simulink model "DiscreteStateSpace"  (R2017a)
settings: Solver=FixedStepAuto  StartTime=0.0  StopTime=10.0  FixedStep=sys.Ts  RelTol=1e-3
undefined symbols (not defined in the file): sys
settings Model: Creator=bhannigan  LastModifiedBy=bhannigan

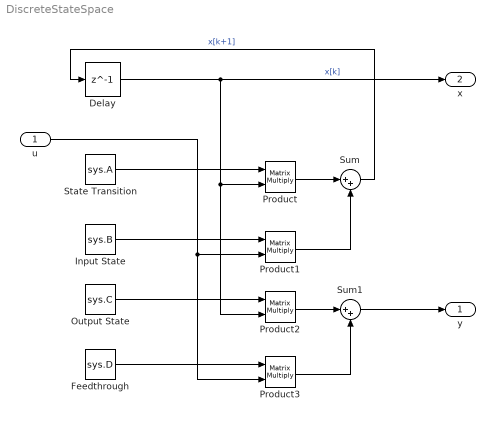
== system DiscreteStateSpace ==
  u : Inport
  Delay : Delay  DelayLength=1  InitialCondition=0
  Feedthrough : Constant  Value=sys.D  VectorParams1D=off
  Input State : Constant  Value=sys.B  VectorParams1D=off
  Output State : Constant  Value=sys.C  VectorParams1D=off
  Product{,1..3} (4 alike) : Product  Multiplication=Matrix(*)
  State Transition : Constant  Value=sys.A  VectorParams1D=off
  Sum : Sum  Inputs=|++
  Sum1 : Sum  Inputs=|++
  y : Outport
  x : Outport  Port=2
  wires:
  Delay/1 -> Product/2, Product2/2, x/1  "x[k]"
  Product/1 -> Sum/1
  Product1/1 -> Sum/2
  Sum/1 -> Delay/1  "x[k+1]"
  Product2/1 -> Sum1/1
  Product3/1 -> Sum1/2
  Sum1/1 -> y/1
  u/1 -> Product1/2, Product3/2
  Feedthrough/1 -> Product3/1
  Output State/1 -> Product2/1
  Input State/1 -> Product1/1
  State Transition/1 -> Product/1
